simulink model "BC_MR"  (R2025b)
settings: Solver=FixedStepAuto  StartTime=0.0  StopTime=15  FixedStep=TsELEC  RelTol=1e-3  EnableMultiTasking=on
InitFcn:
  | TsELEC = Ts;
  | TsMECH = 5e-4;
  | TsTHERMAL = 1e-3;
  | 
  | Ts_speed = 1e-4;
  | Ts_inverter = Ts;
  | Ts_motor = Ts;
  | Ts_simulink = Ts;
  | 
  | 
  | PM = 0.03*10; % Permanent magnet flux linkage
  | Ld = 2e-3;  % d-axis inductance
  | Lq = 2e-3;  % q-axis inductance
  | L0 = 2e-3;  % 0-axis inductance
  | Rs = 0.0013; % Stator resistance
  | N = 2; % Number of pole pairs
  | J = 0.2; % Moment of inertia
values from neighbouring files (symbols this model uses):
  combustor_volume = 0.001    [initParams.mat]
  compressor =     [initParams.mat]
  flow_area = 0.002    [initParams.mat]
  scale_factor = 5    [initParams.mat]
  Ts = 5e-05    [initParams.mat]
  turbine =     [initParams.mat]
undefined symbols (not defined in the file or in its folder): DiscIntNeverNeededParam
libraries: fl_lib x42, nesl_utility x16, BraytonCycle_lib x4
(part 4 of 4)

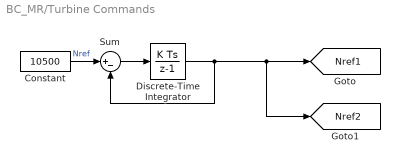
== system BC_MR/Turbine Commands ==
  Constant : Constant  Value=10500  SampleTime=Ts
  Discrete-Time Integrator : DiscreteIntegrator  gainval=1  InitialCondition=10500  SampleTime=TsELEC  ICPrevOutput=DiscIntNeverNeededParam  ICPrevScaledInput=DiscIntNeverNeededParam
  Sum : Sum  Inputs=|+-
  tag scope: Nref1=global, Nref2=global
  wires:
  Discrete-Time Integrator/1 -> [Nref1], [Nref2], Sum/2
  Sum/1 -> Discrete-Time Integrator/1
  Constant/1 -> Sum/1  "Nref"

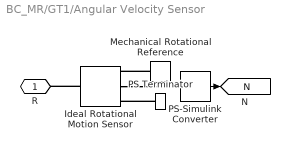
== system BC_MR/GT1/Angular Velocity Sensor ==
  Ideal Rotational Motion Sensor : fl_lib/Mechanical/Mechanical Sensors/Ideal Rotational Motion Sensor  reference=foundation.enum.MeasurementReference.difference  acceleration_port=false  velocity_port=true  position_port=true  wrap_angle=simscape.enum.onoff.off  offset=0 rad
  Mechanical Rotational Reference : fl_lib/Mechanical/Rotational Elements/Mechanical Rotational Reference
  PS Terminator : fl_lib/Physical Signals/Sinks/PS Terminator
  PS-Simulink Converter : nesl_utility/PS-Simulink Converter  PhysicalDomain=network_engine_domain  SubClassName=ps_output  LeftPortType=input  RightPortType=output  PseudoPeriodic=off  Frequencies=[]  VectorFormat=1-D array  Unit=rpm  AffineConversion=off
  R : PMIOPort  Side=Left
  tag scope: N=global
  wires:
  PS-Simulink Converter/1 -> [N]
  connections:
  Ideal Rotational Motion Sensor/LConn1 -- R/RConn1
  Ideal Rotational Motion Sensor/RConn2 -- PS-Simulink Converter/LConn1
  Mechanical Rotational Reference/LConn1 -- Ideal Rotational Motion Sensor/RConn1
  PS Terminator/LConn1 -- Ideal Rotational Motion Sensor/RConn3

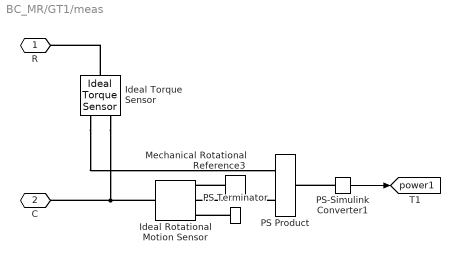
== system BC_MR/GT1/meas ==
  Ideal Rotational Motion Sensor : fl_lib/Mechanical/Mechanical Sensors/Ideal Rotational Motion Sensor  reference=foundation.enum.MeasurementReference.difference  acceleration_port=false  velocity_port=true  position_port=true  wrap_angle=simscape.enum.onoff.off  offset=0 rad
  Ideal Torque Sensor : fl_lib/Mechanical/Mechanical Sensors/Ideal Torque Sensor
  Mechanical Rotational Reference3 : fl_lib/Mechanical/Rotational Elements/Mechanical Rotational Reference
  PS Product : fl_lib/Physical Signals/Functions/PS Product
  PS Terminator : fl_lib/Physical Signals/Sinks/PS Terminator
  PS-Simulink Converter1 : nesl_utility/PS-Simulink Converter  PhysicalDomain=network_engine_domain  SubClassName=ps_output  LeftPortType=input  RightPortType=output  PseudoPeriodic=off  Frequencies=[]  VectorFormat=1-D array  Unit=W  AffineConversion=off
  R : PMIOPort  Side=Right
  C : PMIOPort  Port=2  Side=Left
  tag scope: power1=global
  wires:
  PS-Simulink Converter1/1 -> [power1]
  connections:
  Ideal Torque Sensor/LConn1 -- R/RConn1
  Ideal Torque Sensor/RConn2 -- PS Product/LConn1
  PS Product/LConn2 -- Ideal Rotational Motion Sensor/RConn2
  Ideal Torque Sensor/RConn1 -- C/RConn1 -- Ideal Rotational Motion Sensor/LConn1
  Mechanical Rotational Reference3/LConn1 -- Ideal Rotational Motion Sensor/RConn1
  PS Terminator/LConn1 -- Ideal Rotational Motion Sensor/RConn3
  PS-Simulink Converter1/LConn1 -- PS Product/RConn1

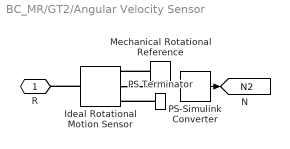
== system BC_MR/GT2/Angular Velocity Sensor ==
  Ideal Rotational Motion Sensor : fl_lib/Mechanical/Mechanical Sensors/Ideal Rotational Motion Sensor  reference=foundation.enum.MeasurementReference.difference  acceleration_port=false  velocity_port=true  position_port=true  wrap_angle=simscape.enum.onoff.off  offset=0 rad
  Mechanical Rotational Reference : fl_lib/Mechanical/Rotational Elements/Mechanical Rotational Reference
  PS Terminator : fl_lib/Physical Signals/Sinks/PS Terminator
  PS-Simulink Converter : nesl_utility/PS-Simulink Converter  PhysicalDomain=network_engine_domain  SubClassName=ps_output  LeftPortType=input  RightPortType=output  PseudoPeriodic=off  Frequencies=[]  VectorFormat=1-D array  Unit=rpm  AffineConversion=off
  R : PMIOPort  Side=Left
  tag scope: N2=global
  wires:
  PS-Simulink Converter/1 -> [N2]
  connections:
  PS Terminator/LConn1 -- Ideal Rotational Motion Sensor/RConn3
  Mechanical Rotational Reference/LConn1 -- Ideal Rotational Motion Sensor/RConn1
  Ideal Rotational Motion Sensor/RConn2 -- PS-Simulink Converter/LConn1
  Ideal Rotational Motion Sensor/LConn1 -- R/RConn1

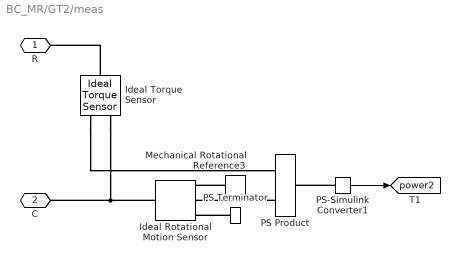
== system BC_MR/GT2/meas ==
  Ideal Rotational Motion Sensor : fl_lib/Mechanical/Mechanical Sensors/Ideal Rotational Motion Sensor  reference=foundation.enum.MeasurementReference.difference  acceleration_port=false  velocity_port=true  position_port=true  wrap_angle=simscape.enum.onoff.off  offset=0 rad
  Ideal Torque Sensor : fl_lib/Mechanical/Mechanical Sensors/Ideal Torque Sensor
  Mechanical Rotational Reference3 : fl_lib/Mechanical/Rotational Elements/Mechanical Rotational Reference
  PS Product : fl_lib/Physical Signals/Functions/PS Product
  PS Terminator : fl_lib/Physical Signals/Sinks/PS Terminator
  PS-Simulink Converter1 : nesl_utility/PS-Simulink Converter  PhysicalDomain=network_engine_domain  SubClassName=ps_output  LeftPortType=input  RightPortType=output  PseudoPeriodic=off  Frequencies=[]  VectorFormat=1-D array  Unit=W  AffineConversion=off
  R : PMIOPort  Side=Right
  C : PMIOPort  Port=2  Side=Left
  tag scope: power2=global
  wires:
  PS-Simulink Converter1/1 -> [power2]
  connections:
  PS-Simulink Converter1/LConn1 -- PS Product/RConn1
  PS Terminator/LConn1 -- Ideal Rotational Motion Sensor/RConn3
  Mechanical Rotational Reference3/LConn1 -- Ideal Rotational Motion Sensor/RConn1
  Ideal Rotational Motion Sensor/LConn1 -- C/RConn1 -- Ideal Torque Sensor/RConn1
  PS Product/LConn2 -- Ideal Rotational Motion Sensor/RConn2
  Ideal Torque Sensor/RConn2 -- PS Product/LConn1
  Ideal Torque Sensor/LConn1 -- R/RConn1
